simulink model "mIntegratedModel"  (R2021b)
settings: Solver=FixedStepDiscrete  StartTime=0.0  StopTime=1  RelTol=1e-3
PreLoadFcn:
  | A=1;B=1;C=2;D=1;
undefined symbols (not defined in the file or in its folder): sigbuilder_block
CloseFcn:
  | clear A B C D;
settings Model: Creator=nrangava  LastModifiedBy=nrangava
settings SolverCC: AlgebraicLoopSolver=TrustRegion  MaxZcPerStep=1
settings DataIOCC: SaveFormat=StructureWithTime  SaveState=on  DSMLogging=off  OutputSaveName=yout1,yout2
settings OptimizationCC: DefaultParameterBehavior=Inlined  EnhancedBackFolding=on  PassReuseOutputArgsAs=Individual arguments  ZeroExternalMemoryAtStartup=off  ZeroInternalMemoryAtStartup=off  OptimizeBlockOrder=speed  DifferentSizesBufferReuse=on  OptimizationCustomize=off  EfficientTunableParamExpr=on
settings DebuggingCC: ParameterTunabilityLossMsg=error  SFMachineParentedDataDiag=warning
settings HardwareCC: TargetBitPerPointer=64  TargetBitPerSizeT=64  TargetBitPerPtrDiffT=64  TargetLongLongMode=on  TargetIntDivRoundTo=Zero  TargetEndianess=LittleEndian  TargetWordSize=64  TargetHWDeviceType=Custom Processor->MATLAB Host Computer  ProdEqTarget=off
settings ModelReferenceCC: UpdateModelReferenceTargets=IfOutOfDate
settings SFSimCC: MATLABDynamicMemAlloc=off
settings RTWCC: Description=Embedded Coder  SystemTargetFile=ert.tlc  TemplateMakefile=ert_default_tmf  RTWVerbose=off  RetainRTWFile=on  TLCAssert=on
settings CodeAppCC: ForceParamTrailComments=on  IgnoreCustomStorageClasses=off  MaxIdLength=64  OperatorAnnotations=on  SimulinkDataObjDesc=on  SFDataObjDesc=on  InsertBlockDesc=on
settings ERTTargetCC: TargetLangStandard=C99 (ISO)  GenerateSampleERTMain=on  CombineOutputUpdateFcns=off  LogVarNameModifier=none  MatFileLogging=on  InlinedParameterPlacement=NonHierarchical  ERTCustomFileTemplate=example_file_process.tlc

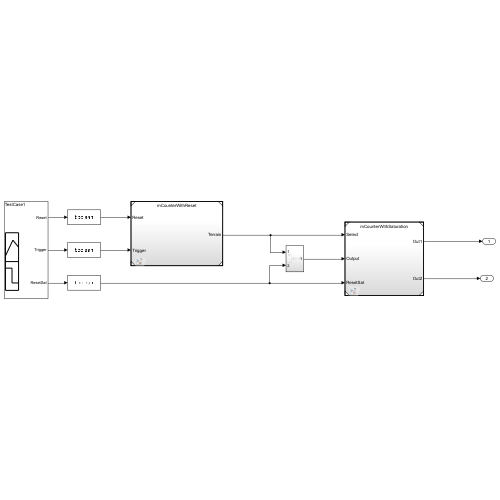
[thumbnail: Simulink's stored preview of the top-level diagram]
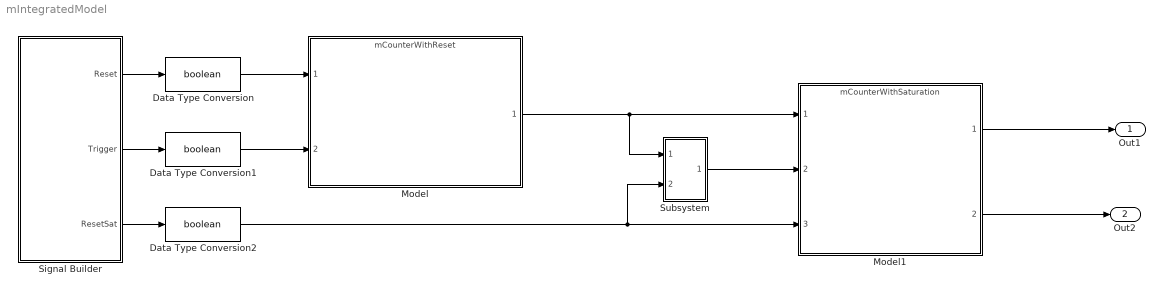
== system mIntegratedModel ==
  Data Type Conversion : DataTypeConversion  OutDataTypeStr=boolean
  Data Type Conversion1 : DataTypeConversion  OutDataTypeStr=boolean
  Data Type Conversion2 : DataTypeConversion  OutDataTypeStr=boolean
  Model : ModelReference  ModelNameDialog=mCounterWithReset.slx  SimulationMode=Normal  ModelReferenceVersion=4.4
  Model1 : ModelReference  ModelNameDialog=mCounterWithSaturation.slx  SimulationMode=Normal  ModelReferenceVersion=4.2
  Signal Builder : Subsystem  Tag=STV Subsys  LoadFcn=sigbuilder_block('load');  StartFcn=sigbuilder_block('start');  StopFcn=sigbuilder_block('stop');  ClipboardFcn=sigbuilder_block('clipboard');  mask(Sigbuilder block){tuvar=[0:10]}
      mask help: Simulink:masks:SigbuilderBlock_MD
      mask init:
      | if ~strcmp(get_param(bdroot(gcbh),'SimulationStatus'),'stopped') tuvar = sigbuilder_block('maskInit'); end
      settings: CopyFcn=sigbuilder_block('copy');  DeleteFcn=sigbuilder_block('delete');  ModelCloseFcn=sigbuilder_block('modelClose');  PreSaveFcn=sigbuilder_block('preSave');  PauseFcn=sigbuilder_block('pause');  ContinueFcn=sigbuilder_block('continue');  NameChangeFcn=sigbuilder_block('namechange');  OpenFcn=sigbuilder_block('open',[393 126.6 550.8 400.2 ]);  CloseFcn=sigbuilder_block('close');
      mask Display: plot(0, 0, 100, 100,[2, 2, 32, 32, 2], [68, 8, 8, 68, 68],[32, 2], [38, 38], [32, 19, 2],[53, 60, 44], [32, 17, 17, 2],[16, 16, 31, 31]);txt = getActiveGroup(gcbh);text(2, 100, txt,'verticalAlignment', 'top');
  Subsystem : Subsystem
  Out1 : Outport
  Out2 : Outport  Port=2
  wires:
  Signal Builder/1(Reset) -> Data Type Conversion/1
  Signal Builder/2(Trigger) -> Data Type Conversion1/1
  Model/1 -> Subsystem/1(In1), Model1/1
  Signal Builder/3(ResetSat) -> Data Type Conversion2/1
  Subsystem/1(Out1) -> Model1/2
  Model1/1 -> Out1/1
  Model1/2 -> Out2/1
  Data Type Conversion/1 -> Model/1
  Data Type Conversion1/1 -> Model/2
  Data Type Conversion2/1 -> Model1/3, Subsystem/2(In2)

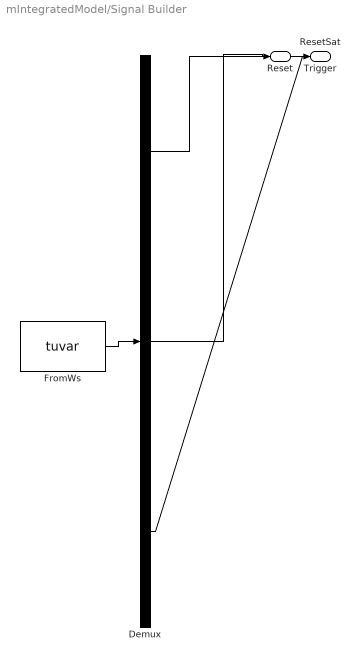
== system mIntegratedModel/Signal Builder ==
  Demux : Demux  Tag=STV Demux  Outputs=3
      settings: DisplayOption=none
  FromWs : FromWorkspace  Tag=STV FromWs  VariableName=tuvar  SampleTime=0.2
      SigBuilderData=|
      | common.afterFinalStr = 'Extrapolate'
      | common.sampleTime = '0.2'
      | dataSet(1).timeRange = [0 1]
      | dataSet(1).name = 'TestCase1'
      | dataSet(2).timeRange = [0 1]
      | dataSet(2).name = 'TestCase2'
      | sbobj.Groups(1).Name = 'TestCase1'
      | sbobj.Groups(1).Signals(1).Name = 'Reset'
      | sbobj.Groups(1).Signals(1).XData = [0 0.2 0.4 0.6 0.8 1]
      | sbobj.Groups(1).Signals(1).YData = [0 0 0 0 0 0]
      | sbobj.Groups(1).Signals(2).Name = 'Trigger'
      | sbobj.Groups(1).Signals(2).XData = [0 0.2 0.4 0.6 0.8 1]
      | sbobj.Groups(1).Signals(2).YData = [1 0 0 1 0 1]
      | sbobj.Groups(1).Signals(3).Name = 'ResetSat'
      | sbobj.Groups(1).Signals(3).XData = [0 0.2 0.4 0.6 0.8 1]
      | sbobj.Groups(1).Signals(3).YData = [0 0 0 0 0 0]
      | sbobj.Groups(1).TimeRange = [0 1]
      | sbobj.Groups(2).Name = 'TestCase2'
      | sbobj.Groups(2).Signals(1).Name = 'Reset'
      | sbobj.Groups(2).Signals(1).XData = [0 0.2 0.4 0.6 0.8 1]
      | sbobj.Groups(2).Signals(1).YData = [1 1 1 0 0 0]
      | sbobj.Groups(2).Signals(2).Name = 'Trigger'
      | sbobj.Groups(2).Signals(2).XData = [0 0.2 0.4 0.6 0.8 1]
      | sbobj.Groups(2).Signals(2).YData = [1 1 1 1 1 1]
      | sbobj.Groups(2).Signals(3).Name = 'ResetSat'
      | sbobj.Groups(2).Signals(3).XData = [0 0.2 0.4 0.6 0.8 1]
      | sbobj.Groups(2).Signals(3).YData = [0 0 0 1 1 1]
      | sbobj.Groups(2).TimeRange = [0 1]
  Reset : Outport  Tag=STV Outport
  Trigger : Outport  Tag=STV Outport  Port=2
  ResetSat : Outport  Tag=STV Outport  Port=3
  wires:
  Demux/1 -> Reset/1
  FromWs/1 -> Demux/1
  Demux/2 -> Trigger/1
  Demux/3 -> ResetSat/1

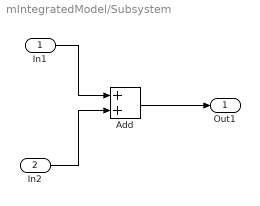
== system mIntegratedModel/Subsystem ==
  In1 : Inport
  In2 : Inport  Port=2
  Add : Sum
  Out1 : Outport
  wires:
  In1/1 -> Add/1
  Add/1 -> Out1/1
  In2/1 -> Add/2
